simulink model "project_two_Abdoul"  (R2017b)
settings: Solver=VariableStepAuto  StartTime=0.0  StopTime=inf  RelTol=1e-3
libraries: libraryProject2 x4, realtime_pacer_lib x1
settings Model: Creator=BRAHIMA FANNY  LastModifiedBy=abdoul kader
settings CodeAppCC: StateflowObjectComments=on

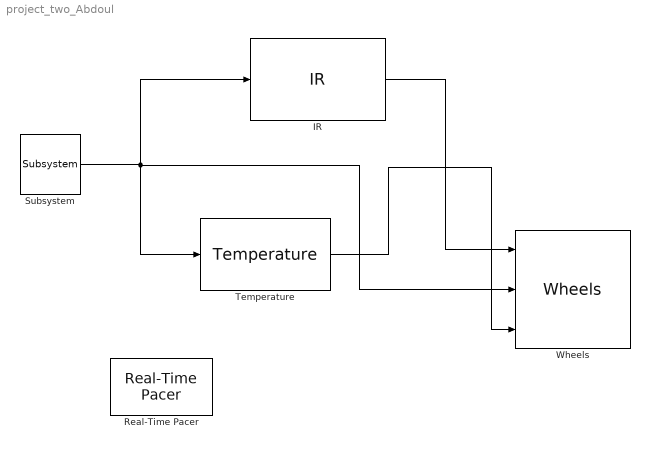
== system project_two_Abdoul ==
  "IR " : libraryProject2/IR 
  Real-Time Pacer : realtime_pacer_lib/Real-Time Pacer  simTimePerRealTime=.5
  Subsystem : libraryProject2/Subsystem
  Temperature : libraryProject2/Temperature
  Wheels : libraryProject2/Wheels
  wires:
  "IR "/1 -> Wheels/1
  Temperature/1 -> Wheels/3
  Subsystem/1 -> Wheels/2, Temperature/1, "IR "/1
